simulink model "table_23_scenario_2"  (R2023b)
settings: Solver=VariableStepAuto  StartTime=0.0  StopTime=20.0  RelTol=1e-3
undefined symbols (not defined in the file or in its folder): sigbuilder_block
libraries: fuzblock x1
settings Model: Creator=User  LastModifiedBy=user
settings DebuggingCC: UnconnectedInputMsg=warning  UnconnectedOutputMsg=warning  UnconnectedLineMsg=warning
settings ModelReferenceCC: EnableRefExpFcnMdlSchedulingChecks=on
settings RTWCC: DLArmComputeVersion=19.05

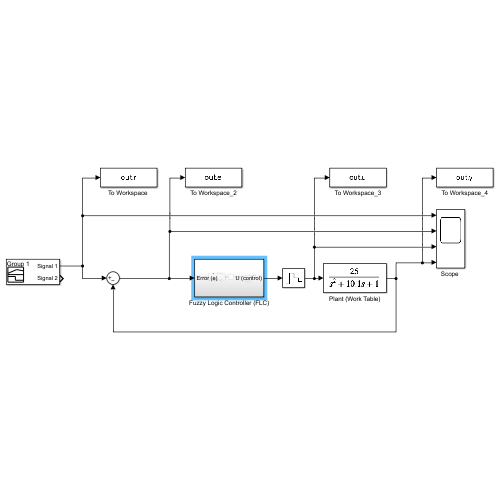
[thumbnail: Simulink's stored preview of the top-level diagram]
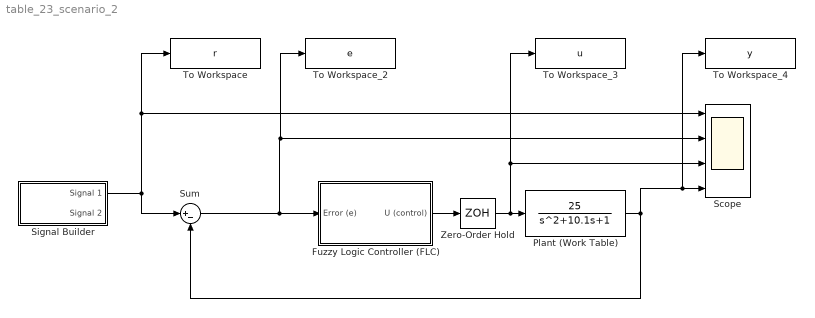
== system table_23_scenario_2 ==
  Fuzzy Logic Controller (FLC) : Subsystem
  Plant (Work Table) : TransferFcn  Numerator=[25]  Denominator=[1 10.1 1]
  "Scope " : Scope  NumInputPorts=4
  Signal Builder : Subsystem  Tag=STV Subsys  LoadFcn=sigbuilder_block('load');  StartFcn=sigbuilder_block('start');  StopFcn=sigbuilder_block('stop');  ClipboardFcn=sigbuilder_block('clipboard');  mask(Sigbuilder block){tuvar=[0:10]}
      mask help: Simulink:masks:SigbuilderBlock_MD
      mask init:
      | if ~strcmp(get_param(bdroot(gcbh),'SimulationStatus'),'stopped') tuvar = sigbuilder_block('maskInit'); end
      settings: CopyFcn=sigbuilder_block('copy');  DeleteFcn=sigbuilder_block('delete');  ModelCloseFcn=sigbuilder_block('modelClose');  PreSaveFcn=sigbuilder_block('preSave');  PauseFcn=sigbuilder_block('pause');  ContinueFcn=sigbuilder_block('continue');  NameChangeFcn=sigbuilder_block('namechange');  OpenFcn=sigbuilder_block('open',[5.4 36 1141.2 516.6 ]);  CloseFcn=sigbuilder_block('close');
      mask Display: plot(0, 0, 100, 100,[2, 2, 32, 32, 2], [68, 8, 8, 68, 68],[32, 2], [38, 38], [32, 19, 2],[53, 60, 44], [32, 17, 17, 2],[16, 16, 31, 31]);txt = getActiveGroup(gcbh);text(2, 100, txt,'verticalAlignment', 'top');
  Sum : Sum  Inputs=|+-
  "To Workspace " : ToWorkspace  VariableName=r  SaveFormat=Timeseries  SampleTime=-1
  To Workspace_2 : ToWorkspace  VariableName=e  SaveFormat=Timeseries  SampleTime=-1
  To Workspace_3 : ToWorkspace  VariableName=u  SaveFormat=Timeseries  SampleTime=-1
  To Workspace_4 : ToWorkspace  VariableName=y  SaveFormat=Timeseries  SampleTime=-1
  Zero-Order Hold : ZeroOrderHold  SampleTime=-1
  wires:
  Plant (Work Table)/1 -> To Workspace_4/1, "Scope "/4, Sum/2
  Sum/1 -> To Workspace_2/1, "Scope "/2, Fuzzy Logic Controller (FLC)/1(Error (e))
  Fuzzy Logic Controller (FLC)/1("\tU (control)") -> Zero-Order Hold/1
  Zero-Order Hold/1 -> To Workspace_3/1, "Scope "/3, Plant (Work Table)/1
  Signal Builder/1(Signal 1) -> Sum/1, "Scope "/1, "To Workspace "/1

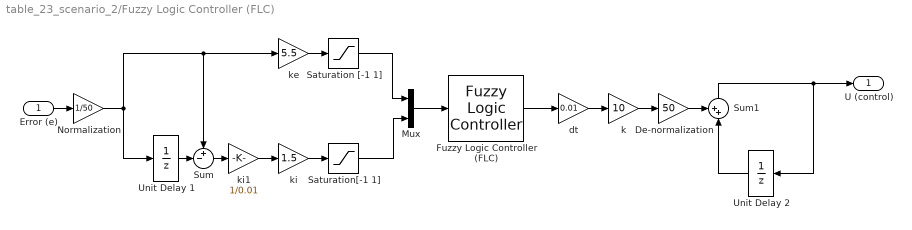
== system table_23_scenario_2/Fuzzy Logic Controller (FLC) ==
  Error (e) : Inport
  De-normalization : Gain  Gain=50
  Fuzzy Logic Controller (FLC) : fuzblock/Fuzzy Logic  Controller  FIS=fis_table_23  OutputSampleNumber=101  DataType=double  FuzzifiedInputs=off  RuleFiringStrengths=off  RuleOutputs=off  AggregatedOutputs=off  SimulateUsing=Interpreted execution  OutOfRangeInputValueMessage=warning  NoRuleFiredMessage=warning  EmptyOutputFuzzySetMessage=warning
  Mux : Mux  Inputs=2
  Normalization : Gain  Gain=1/50
  Saturation [-1 1] : Saturate  UpperLimit=1  LowerLimit=-1
  "Saturation[-1 1] " : Saturate  UpperLimit=1  LowerLimit=-1
  Sum : Sum  Inputs=+-|
  Sum1 : Sum  Inputs=++|
  Unit Delay 1 : UnitDelay  SampleTime=0.01  HasFrameUpgradeWarning=on
  Unit Delay 2 : UnitDelay  SampleTime=0.01  HasFrameUpgradeWarning=on
  dt : Gain  Gain=0.01
  k : Gain  Gain=10
  ke : Gain  Gain=5.5
  ki : Gain  Gain=1.5
  ki1 : Gain  Gain=1/0.01
  "\tU (control)" : Outport
  wires:
  Error (e)/1 -> Normalization/1
  Fuzzy Logic Controller (FLC)/1 -> dt/1
  Mux/1 -> Fuzzy Logic Controller (FLC)/1
  ki1/1 -> ki/1
  ke/1 -> Saturation [-1 1]/1
  Normalization/1 -> Unit Delay 1/1, Sum/1, ke/1
  Saturation [-1 1]/1 -> Mux/1
  "Saturation[-1 1] "/1 -> Mux/2
  Unit Delay 1/1 -> Sum/2
  Sum/1 -> ki1/1
  De-normalization/1 -> Sum1/1
  Unit Delay 2/1 -> Sum1/2
  ki/1 -> "Saturation[-1 1] "/1
  dt/1 -> k/1
  k/1 -> De-normalization/1
  Sum1/1 -> Unit Delay 2/1, "\tU (control)"/1

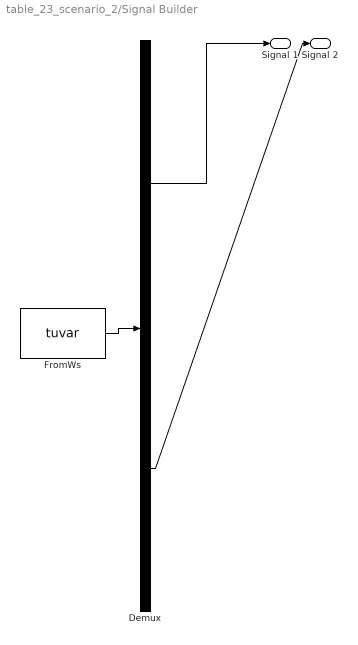
== system table_23_scenario_2/Signal Builder ==
  Demux : Demux  Tag=STV Demux  Outputs=2
      settings: DisplayOption=none
  FromWs : FromWorkspace  Tag=STV FromWs  VariableName=tuvar
      SigBuilderData=|
      | common.afterFinalStr = 'Extrapolate'
      | common.sampleTime = 0
      | dataSet.timeRange = [0 20]
      | dataSet.name = 'Group 1'
      | sbobj.Groups.Name = 'Group 1'
      | sbobj.Groups.Signals(1).Name = 'Signal 1'
      | sbobj.Groups.Signals(1).XData = [0 5 5 10 10 20]
      | sbobj.Groups.Signals(1).YData = [50 50 20 20 40 40]
      | sbobj.Groups.Signals(2).Name = 'Signal 2'
      | sbobj.Groups.Signals(2).XData = [0 5 10 20]
      | sbobj.Groups.Signals(2).YData = [0.4 50 50 0.4]
      | sbobj.Groups.TimeRange = [0 20]
  Signal 1 : Outport  Tag=STV Outport
  Signal 2 : Outport  Tag=STV Outport  Port=2
  wires:
  Demux/1 -> Signal 1/1
  FromWs/1 -> Demux/1
  Demux/2 -> Signal 2/1
